simulink model "GradingSys"  (R2018b)
settings: Solver=VariableStepAuto  StartTime=0.0  StopTime=10  RelTol=1e-3
settings Model: Creator=lenovo2  LastModifiedBy=lenovo2

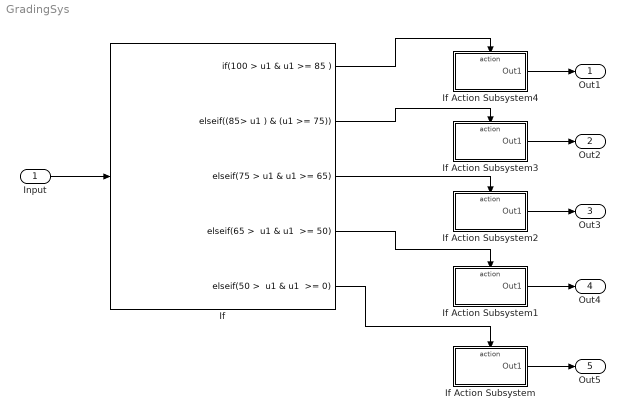
== system GradingSys ==
  Input : Inport
  If : If  IfExpression=100 > u1 & u1 >= 85  ElseIfExpressions="(85> u1 ) & (u1 >= 75), 75 > u1 & u1 >= 65, 65 >  u1 & u1  >= 50, 50 >  u1 & u1  >= 0"  ShowElse=off
  If Action Subsystem : Subsystem  TreatAsAtomicUnit=on
  If Action Subsystem1 : Subsystem  TreatAsAtomicUnit=on
  If Action Subsystem2 : Subsystem  TreatAsAtomicUnit=on
  If Action Subsystem3 : Subsystem  TreatAsAtomicUnit=on
  If Action Subsystem4 : Subsystem  TreatAsAtomicUnit=on
  Out1 : Outport
  Out2 : Outport  Port=2
  Out3 : Outport  Port=3
  Out4 : Outport  Port=4
  Out5 : Outport  Port=5
  wires:
  Input/1 -> If/1
  If/1 -> If Action Subsystem4/Action
  If/2 -> If Action Subsystem3/Action
  If/3 -> If Action Subsystem2/Action
  If/4 -> If Action Subsystem1/Action
  If/5 -> If Action Subsystem/Action
  If Action Subsystem4/1(Out1) -> Out1/1
  If Action Subsystem3/1(Out1) -> Out2/1
  If Action Subsystem2/1(Out1) -> Out3/1
  If Action Subsystem1/1(Out1) -> Out4/1
  If Action Subsystem/1(Out1) -> Out5/1

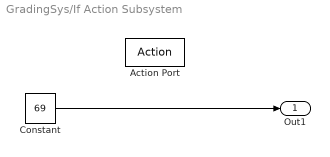
== system GradingSys/If Action Subsystem ==
  Action Port : ActionPort  ActionType=elseif
  Constant : Constant  Value=69
  Out1 : Outport
  wires:
  Constant/1 -> Out1/1

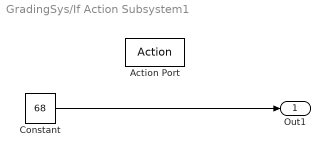
== system GradingSys/If Action Subsystem1 ==
  Action Port : ActionPort  ActionType=elseif
  Constant : Constant  Value=68
  Out1 : Outport
  wires:
  Constant/1 -> Out1/1

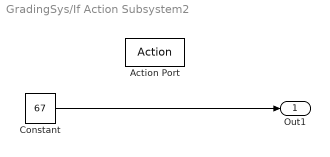
== system GradingSys/If Action Subsystem2 ==
  Action Port : ActionPort  ActionType=elseif
  Constant : Constant  Value=67
  Out1 : Outport
  wires:
  Constant/1 -> Out1/1

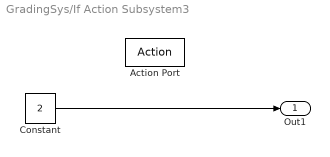
== system GradingSys/If Action Subsystem3 ==
  Action Port : ActionPort  ActionType=elseif
  Constant : Constant  Value=2
  Out1 : Outport
  wires:
  Constant/1 -> Out1/1

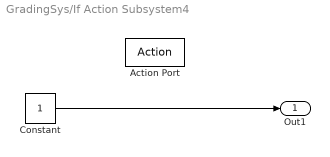
== system GradingSys/If Action Subsystem4 ==
  Action Port : ActionPort  ActionType=then
  Constant : Constant
  Out1 : Outport
  wires:
  Constant/1 -> Out1/1
